simulink model "car_model"  (Simulink 7.5)
settings: Solver=ode45  StartTime=0.0  StopTime=10.0  RelTol=1e-3
undefined symbols (not defined in the file or in its folder): f_F0, f_R0, u0, X0
settings Model: Creator=oktay  LastModifiedBy=oktay

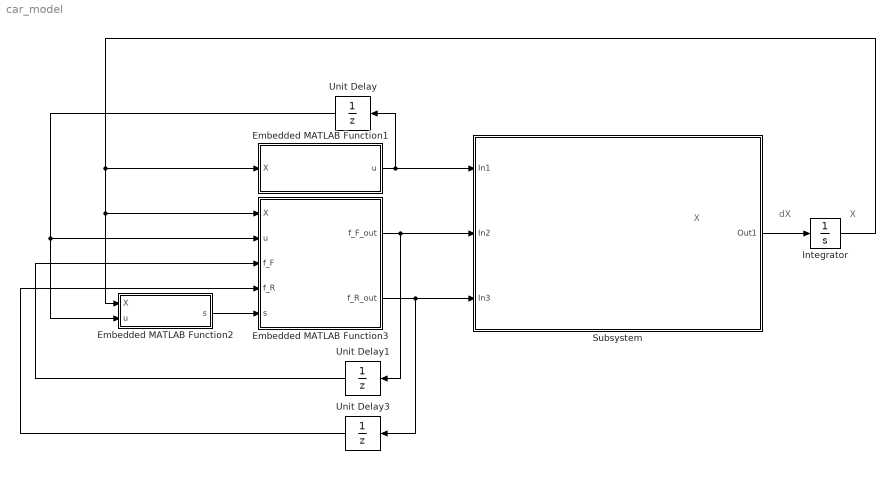
== system car_model ==
  note: X
  note: dX
  note: X
  Embedded MATLAB Function1 : Stateflow chart  TreatAsAtomicUnit=on
  Embedded MATLAB Function2 : Stateflow chart  TreatAsAtomicUnit=on
  Embedded MATLAB Function3 : Stateflow chart  TreatAsAtomicUnit=on
  Integrator : Integrator  InitialCondition=X0
  Subsystem : Subsystem
      mask Display: image(imread('car_logo.png'))
  Unit Delay : UnitDelay  X0=u0  SampleTime=-1
  Unit Delay1 : UnitDelay  X0=f_F0  SampleTime=-1
  Unit Delay3 : UnitDelay  X0=f_R0  SampleTime=-1
  wires:
  Subsystem/1(Out1) -> Integrator/1
  Embedded MATLAB Function3/1(f_F_out) -> Unit Delay1/1, Subsystem/2(In2)
  Embedded MATLAB Function3/2(f_R_out) -> Subsystem/3(In3), Unit Delay3/1
  Embedded MATLAB Function1/1(u) -> Unit Delay/1, Subsystem/1(In1)
  Embedded MATLAB Function2/1(s) -> Embedded MATLAB Function3/5(s)
  Integrator/1 -> Embedded MATLAB Function1/1(X), Embedded MATLAB Function2/1(X), Embedded MATLAB Function3/1(X)
  Unit Delay/1 -> Embedded MATLAB Function2/2(u), Embedded MATLAB Function3/2(u)
  Unit Delay1/1 -> Embedded MATLAB Function3/3(f_F)
  Unit Delay3/1 -> Embedded MATLAB Function3/4(f_R)

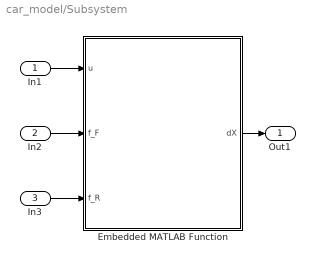
== system car_model/Subsystem ==
  In1 : Inport
  In2 : Inport  Port=2
  In3 : Inport  Port=3
  Embedded MATLAB Function : Stateflow chart  TreatAsAtomicUnit=on
  Out1 : Outport
  wires:
  In1/1 -> Embedded MATLAB Function/1(u)
  In2/1 -> Embedded MATLAB Function/2(f_F)
  In3/1 -> Embedded MATLAB Function/3(f_R)
  Embedded MATLAB Function/1(dX) -> Out1/1

== matlab function Embedded MATLAB Function1 ==
  data: u output double; X input double
function u = controller(X)
%#eml

f_Fx = 0;
f_Rx = 0;
delta = 0;

u = [f_Fx, f_Rx, delta];

== matlab function Subsystem/Embedded MATLAB Function ==
  data: u input double; f_F input double; f_R input double; dX output double
function dX = car_dynamics(u, f_F, f_R)
%#eml

m = param.m;
Iz = param.Iz;
l_F = param.l_F;
l_R = param.l_R;
B = param.B;
C = param.C;
mu = param.mu;
delta_max = param.delta_max;

f_Fx  = u(1);
f_Rx  = u(2);
delta = u(3);

f_Fy = f_F(1);
f_Fz = f_F(2);

f_Ry = f_R(1);
f_Rz = f_R(2);


dVx = 1/m*(f_Fx*cos(delta) - f_Fy*sin(delta) + f_Rx) + Vy*r;
dVy = 1/m*(f_Fx*sin(delta) + f_Fy*cos(delta) + f_Ry) - Vx*r;
dr = 1/Iz*((f_Fy*cos(delta) + f_Fx*sin(delta))*l_F - f_Ry*l_R);
dpsi = r; 

dX = [dVx dVy dr dpsi];

== matlab function Embedded MATLAB Function2 ==
  data: X input double; s output double; u input double
function s = lateral_slips(X, u)
%#eml

l_F = param.l_F;
l_R = param.l_R;

Vx  = X(1);
Vy  = X(2);
r   = X(3);
psi = X(4); 

f_Fx  = u(1);
f_Rx  = u(2);
delta = u(3);


beta = atan(Vy/Vx);
V = sqrt(Vx^2 + Vy^2);

s_Fy = (V*sin(beta-delta) + r*l_F*cos(delta))/(V*cos(beta-delta) + r*l_F*sin(delta));
s_Ry = (V*sin(beta) - r*l_R)/(V*cos(beta));

s = [s_Fy, s_Ry];

== matlab function Embedded MATLAB Function3 ==
  data: f_F_out output double; f_R_out output double; X input double; u input double; f_F input double; f_R input double; s input double
function [f_F_out, f_R_out] = forces (X, u, f_F, f_R, s)

m = param.m;
l_F = param.l_F;
l_R = param.l_R;
mu = param.mu;

Vx  = X(1); 
Vy  = X(2);
r   = X(3);
psi = X(4);

f_Fx  = u(1);
f_Rx  = u(2);
delta = u(3);

f_Fy = f_F(1);  
f_Fz = f_F(2);

f_Ry = f_R(1);  
f_Rz = f_R(2);

s_Fy = s(1);
s_Ry = s(2); 


f_Fz_out = m*g*l_R*(l_F + l_R);
f_Rz_out = m*g*l_F*(l_F + l_R);

f_Fy_max = sqrt((mu*f_Fz)^2 - f_Fx^2);
f_Ry_max = sqrt((mu*f_Rz)^2 - f_Rx^2);

f_Fy_out = f_Fy_max*sin(C*atan(B*s_Fy)); 
f_Ry_out = f_Ry_max*sin(C*atan(B*s_Ry));

f_F_out = [f_Fy_out, f_Fz_out];
f_R_out = [f_Ry_out, f_Rz_out];
